simulink model "CementPlantVer1"  (R2019b)
settings: Solver=ode4  StartTime=0.0  StopTime=inf  FixedStep=0.01  RelTol=1e-3
(part 1 of 2)
settings Model: EnablePacing=on  Creator=huynh  LastModifiedBy=huynh

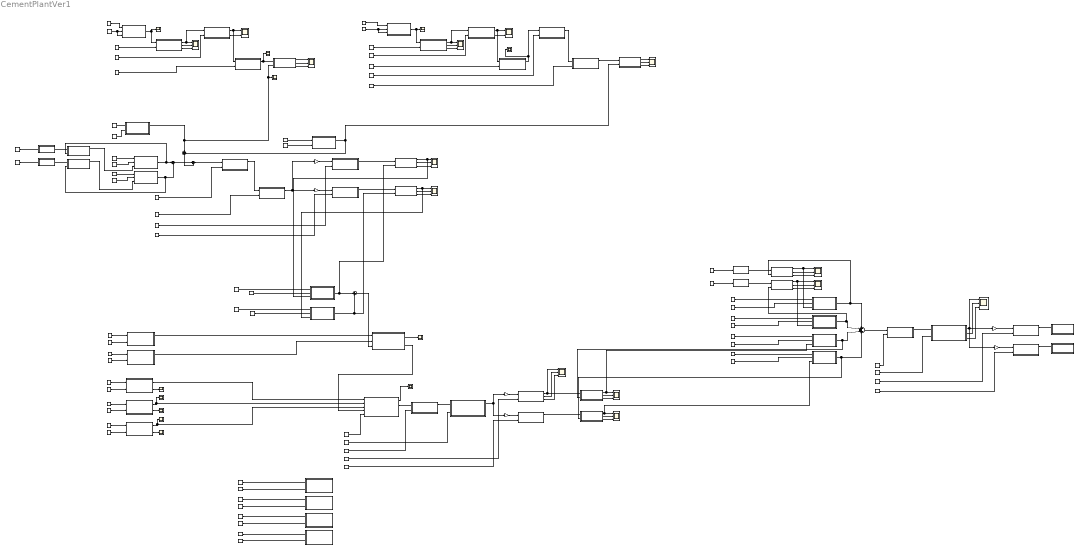
== system CementPlantVer1 ==
  note: CLAY AREA
  note: CementMill
  note: Fan System
  note: Clinker Area
  note: CoalMill
  note: RawMill
  note: Limestone Area
  note: Clay Area
  note: LIMESTONE AREA
  note: RAW MILL
  note: COAL MILL
  note: CLINKER AREA
  note: CEMENT MILL
  Additives Silo : Subsystem  mask{DensityOfMaterial=2.74, HighLevelSet=18, LowLevelSet=5, OutputGain=2}
      mask prompts: DensityOfMaterial "Density of material"; HighLevelSet "High Level"; LowLevelSet "Low Level"; OutputGain "Output Gain"
  Cement Silo 1 : Subsystem  mask{DensityOfMaterial=2.74, HighLevelSet=18, LowLevelSet=5, OutputGain=2}
      mask prompts: DensityOfMaterial "Density of material"; HighLevelSet "High Level"; LowLevelSet "Low Level"; OutputGain "Output Gain"
  Cement Silo 2 : Subsystem  mask{DensityOfMaterial=2.74, HighLevelSet=18, LowLevelSet=5, OutputGain=2}
      mask prompts: DensityOfMaterial "Density of material"; HighLevelSet "High Level"; LowLevelSet "Low Level"; OutputGain "Output Gain"
  CementMill Additives Valve In : Subsystem  mask{FlowConstant=400}
      mask prompts: FlowConstant "Flow Value"
  CementMill Additives Valve In Control : Constant
  CementMill Additives Valve Out : Subsystem  mask{OutputGain=100}
      mask prompts: OutputGain "Output Gian"
  CementMill Clinker Valve Out 1 : Subsystem  mask{OutputGain=200}
      mask prompts: OutputGain "Output Gian"
  CementMill Clinker Valve Out 2 : Subsystem  mask{OutputGain=200}
      mask prompts: OutputGain "Output Gian"
  CementMill Conveyor 1 : Subsystem
  CementMill Conveyor 2 : Subsystem
  CementMill Conveyor 3 : Subsystem
  CementMill Gypsum Valve In : Subsystem  mask{FlowConstant=400}
      mask prompts: FlowConstant "Flow Value"
  CementMill Gypsum Valve In Control : Constant
  CementMill Gypsum Valve Out : Subsystem  mask{OutputGain=100}
      mask prompts: OutputGain "Output Gian"
  CementMill Mix and Crusher : Subsystem
  Clay Conveyor 1 : Subsystem
  Clay Conveyor 2 : Subsystem
  Clay Crusher 1 : Subsystem
  Clay Storage : Subsystem  mask{DensityOfMaterial=2.74, HighLevelSet=18, LowLevelSet=5, OutputGain=2}
      mask prompts: DensityOfMaterial "Density of material"; HighLevelSet "High Level"; LowLevelSet "Low Level"; OutputGain "Output Gain"
  Clay Valve 1 : Subsystem  mask{OutputGain=400}
      mask prompts: OutputGain "Output Gian"
  Clinker Conveyor 1 : Subsystem
  Clinker Conveyor 2 : Subsystem
  Clinker Conveyor 3 : Subsystem
  Clinker Cooling Crusher : Subsystem
  Clinker Fan 1 : Subsystem
  Clinker Fan 2 : Subsystem
  Clinker Fan 3 : Subsystem
  Clinker Fan 4 : Subsystem
  Clinker In Valve 1 : Subsystem  mask{OutputGain=100}
      mask prompts: OutputGain "Output Gian"
  Clinker In Valve 2 : Subsystem  mask{OutputGain=100}
      mask prompts: OutputGain "Output Gian"
  Clinker PreHeater System : Subsystem
  Clinker PreHeater Temperature : Scope
  Clinker Rotary Kiln : Subsystem
  Clinker Rotary Kiln Temperature : Scope
  Clinker Silo 1 : Subsystem  mask{DensityOfMaterial=2.74, HighLevelSet=18, LowLevelSet=5, OutputGain=2}
      mask prompts: DensityOfMaterial "Density of material"; HighLevelSet "High Level"; LowLevelSet "Low Level"; OutputGain "Output Gain"
  Clinker Silo 2 : Subsystem  mask{DensityOfMaterial=2.74, HighLevelSet=18, LowLevelSet=5, OutputGain=2}
      mask prompts: DensityOfMaterial "Density of material"; HighLevelSet "High Level"; LowLevelSet "Low Level"; OutputGain "Output Gain"
  Clinker Valve Enable 1 : Constant
  Clinker Valve Enable 2 : Constant
  CoalMill Fan 1 : Subsystem
  CoalMill Pump 1 : Subsystem
  CoalMill Pump 2 : Subsystem
  CoalMill Pump 3 : Subsystem
  CoalMill Pump 4 : Subsystem
  Enable {1,3,7,9} (4 alike) : Constant
  Enable 5 : Constant  Value=0
  Enable CementMill Additives Valve Out : Constant
  Enable CementMill Clinker Valve Out 1 : Constant
  Enable CementMill Clinker Valve Out 2 : Constant  Value=0
  Enable CementMill Gypsum Valve Out : Constant
  Enable Clay Valve 1 : Constant
  Enable Clinker Fan {1..4} (4 alike) : Constant
  Enable Iron Valve 1 : Constant
  Enable Limestone Valve 1 : Constant
  Enable RawMill Conveyor 1 : Constant
  Enable RawMill Conveyor 2 : Constant
  Enable Sand Valve 1 : Constant
  F Input {1..5} (5 alike) : Constant  Value=50
  Frequence FB 1 : Scope
  Frequence FB 2 : Scope
  Frequence FB 3 : Scope
  Frequence In Clay Conveyor 1 : Constant  Value=50
  Frequence In Clay Conveyor 2 : Constant  Value=50
  Frequence In Clay Crusher 1 : Constant  Value=50
  Frequence In Limestone Conveyor 1 : Constant  Value=50
  Frequence In Limestone Conveyor 2 : Constant  Value=50
  Frequence In Limestone Conveyor 3 : Constant  Value=50
  Frequence In Limestone Crusher 1 : Constant  Value=50
  Frequence In Limestone Crusher 2 : Constant  Value=50
  Frequency In CementMill Conveyor 1 : Constant  Value=50
  Frequency In CementMill Conveyor 2 : Constant  Value=50
  Frequency In CementMill Conveyor 3 : Constant  Value=50
  Frequency In CementMill Mix and Crusher : Constant  Value=50
  Frequency In Clinker Conveyor 1 : Constant  Value=50
  Frequency In Clinker Conveyor 2 : Constant  Value=50
  Frequency In Clinker Conveyor 3 : Constant  Value=50
  Frequency In Clinker Cooling Crusher : Constant  Value=50
  Frequency In Clinker Fan {1..4} (4 alike) : Constant  Value=50
  Frequency In Clinker Rotary Kiln Frequence : Constant  Value=50
  Frequency In RawMill Conveyor {1..4} (4 alike) : Constant  Value=50
  Frequency In Roller Mill 1 : Constant  Value=50
  Gain{,1..5} (6 alike) : Gain  Gain=0.5
  Gypsum Silo : Subsystem  mask{DensityOfMaterial=2.74, HighLevelSet=18, LowLevelSet=5, OutputGain=2}
      mask prompts: DensityOfMaterial "Density of material"; HighLevelSet "High Level"; LowLevelSet "Low Level"; OutputGain "Output Gain"
  Input Frequency RawMill Conveyor 2 : Constant  Value=50
  Iron Silo : Subsystem  mask{DensityOfMaterial=2.74, HighLevelSet=18, LowLevelSet=5, OutputGain=2}
      mask prompts: DensityOfMaterial "Density of material"; HighLevelSet "High Level"; LowLevelSet "Low Level"; OutputGain "Output Gain"
  Limestone Conveyor 1 : Subsystem
  Limestone Conveyor 2 : Subsystem
  Limestone Conveyor 3 : Subsystem
  Limestone Crusher 1 : Subsystem
  Limestone Crusher 2 : Subsystem
  Limestone Storage : Subsystem  mask{DensityOfMaterial=2.74, HighLevelSet=18, LowLevelSet=5, OutputGain=2}
      mask prompts: DensityOfMaterial "Density of material"; HighLevelSet "High Level"; LowLevelSet "Low Level"; OutputGain "Output Gain"
  Limestone Valve 1 : Subsystem  mask{OutputGain=400}
      mask prompts: OutputGain "Output Gian"
  Output Test 2 : Scope
  Output Test 3 : Scope
  Percent Open CementMill Additives Valve Out : Constant  Value=100
  Percent Open CementMill Clinker Valve Out 1 : Constant  Value=100
  Percent Open CementMill Clinker Valve Out 2 : Constant  Value=100
  Percent Open CementMill Gypsum Valve Out : Constant  Value=100
  Percent Open Clay Valve 1 : Constant  Value=100
  Percent Open Clinker Valve 1 : Constant  Value=100
  Percent Open Clinker Valve 2 : Constant  Value=100
  Percent Open Iron Valve 1 : Constant  Value=100
  Percent Open Limestone Valve 1 : Constant  Value=100
  Percent Open Sand Valve 1 : Constant  Value=100
  RawMill Conveyor 1 : Subsystem  mask{OutputGain=100}
      mask prompts: OutputGain "Output Gain"
  RawMill Conveyor 2 : Subsystem  mask{OutputGain=100}
      mask prompts: OutputGain "Output Gain"
  RawMill Conveyor 3 : Subsystem
  RawMill Conveyor 4 : Subsystem
  RawMill Conveyor 5 : Subsystem
  RawMill Iron Valve In : Subsystem  mask{FlowConstant=300}
      mask prompts: FlowConstant "Flow Value"
  RawMill Iron Valve In Control : Constant
  RawMill Iron Valve Out : Subsystem  mask{OutputGain=100}
      mask prompts: OutputGain "Output Gian"
  RawMill Sand Valve In : Subsystem  mask{FlowConstant=300}
      mask prompts: FlowConstant "Flow Value"
  RawMill Sand Valve In Control : Constant
  RawMill Sand Valve Out : Subsystem  mask{OutputGain=100}
      mask prompts: OutputGain "Output Gian"
  RawMill Silo 1 : Subsystem  mask{DensityOfMaterial=2.74, HighLevelSet=18, LowLevelSet=5, OutputGain=2}
      mask prompts: DensityOfMaterial "Density of material"; HighLevelSet "High Level"; LowLevelSet "Low Level"; OutputGain "Output Gain"
  RawMill Silo 2 : Subsystem  mask{DensityOfMaterial=2.74, HighLevelSet=18, LowLevelSet=5, OutputGain=2}
      mask prompts: DensityOfMaterial "Density of material"; HighLevelSet "High Level"; LowLevelSet "Low Level"; OutputGain "Output Gain"
  Roller Mill 1 : Subsystem
  Sand Silo : Subsystem  mask{DensityOfMaterial=2.74, HighLevelSet=18, LowLevelSet=5, OutputGain=2}
      mask prompts: DensityOfMaterial "Density of material"; HighLevelSet "High Level"; LowLevelSet "Low Level"; OutputGain "Output Gain"
  Scope{1,3..4,6,9,11,13..18} (12 alike) : Scope  NumInputPorts=3
  Scope10 : Scope  NumInputPorts=2
  Scope12 : Scope
  Scope5 : Scope  NumInputPorts=2
  Scope7 : Scope
  Scope8 : Scope
  Sum{,1..3} (4 alike) : Sum  Inputs=|++
  Sum4 : Sum  Inputs=4
  Tốc độ đầu ra1 : Scope
  Tốc độ đầu ra2 : Scope
  wires:
  F Input 1/1 -> CoalMill Pump 1/1(Input Frequence)
  CoalMill Pump 1/2(Output Frequence) -> Frequence FB 1/1
  Enable 1/1 -> CoalMill Pump 1/2(Motor Enable)
  Enable RawMill Conveyor 1/1 -> RawMill Conveyor 1/2(Enable)
  Frequency In RawMill Conveyor 1/1 -> RawMill Conveyor 1/1(Input Frequence)
  RawMill Conveyor 1/1(Flow) -> Sum2/1, Clay Storage/2(Qout), Scope8/1
  F Input 2/1 -> CoalMill Pump 2/1(Input Frequence)
  CoalMill Pump 2/2(Output Frequence) -> Frequence FB 2/1
  CoalMill Pump 2/1(Output RPM) -> Tốc độ đầu ra1/1, Clinker Rotary Kiln/2(RPM In 2)
  Enable 3/1 -> CoalMill Pump 2/2(Motor Enable)
  Enable 5/1 -> CoalMill Pump 3/2(Motor Enable)
  CoalMill Pump 3/2(Output Frequence) -> Frequence FB 3/1
  CoalMill Pump 3/1(Output RPM) -> Clinker Rotary Kiln/3(RPM In 3), Tốc độ đầu ra2/1
  F Input 3/1 -> CoalMill Pump 3/1(Input Frequence)
  Percent Open Clay Valve 1/1 -> Clay Valve 1/1(Opening Percent)
  Enable Clay Valve 1/1 -> Clay Valve 1/3(Level of Silo), Clay Valve 1/2(Enable)
  Clay Valve 1/1(Flow) -> Clay Conveyor 1/1(Flow In), Output Test 2/1
  Frequence In Clay Conveyor 1/1 -> Clay Conveyor 1/2(Frequence In)
  Clay Conveyor 1/2(RPM out) -> Scope4/2
  Clay Conveyor 1/3(Frequence FB) -> Scope4/3
  Frequence In Clay Crusher 1/1 -> Clay Crusher 1/2(Frequence In)
  Clay Conveyor 1/1(Flow out) -> Clay Crusher 1/1(Flow In), Scope4/1
  Clay Crusher 1/1(Flow out) -> Clay Conveyor 2/1(Flow In), Scope5/1
  Clay Crusher 1/2(Frequence FB) -> Scope5/2
  Frequence In Clay Conveyor 2/1 -> Clay Conveyor 2/2(Frequence In)
  Clay Conveyor 2/1(Flow out) -> Scope7/1, Clay Storage/1(Qin)
  Clay Storage/3(Low) -> Scope6/3
  Clay Storage/2(High) -> Scope6/2
  Clay Storage/1(Level) -> Scope6/1
  Enable Limestone Valve 1/1 -> Limestone Valve 1/3(Level of Silo), Limestone Valve 1/2(Enable)
  Limestone Conveyor 1/2(RPM out) -> Scope9/2
  Limestone Storage/3(Low) -> Scope11/3
  Limestone Storage/1(Level) -> Scope11/1
  Frequence In Limestone Crusher 1/1 -> Limestone Crusher 1/2(Frequence In)
  Limestone Crusher 1/1(Flow out) -> Limestone Conveyor 2/1(Flow In), Scope10/1
  Limestone Crusher 1/2(Frequence FB) -> Scope10/2
  Limestone Storage/2(High) -> Scope11/2
  Limestone Valve 1/1(Flow) -> Limestone Conveyor 1/1(Flow In), Output Test 3/1
  Frequence In Limestone Conveyor 1/1 -> Limestone Conveyor 1/2(Frequence In)
  Limestone Conveyor 2/1(Flow out) -> Limestone Crusher 2/1(Flow In), Scope12/1
  Limestone Conveyor 1/3(Frequence FB) -> Scope9/3
  Limestone Conveyor 1/1(Flow out) -> Limestone Crusher 1/1(Flow In), Scope9/1
  Percent Open Limestone Valve 1/1 -> Limestone Valve 1/1(Opening Percent)
  Frequence In Limestone Conveyor 2/1 -> Limestone Conveyor 2/2(Frequence In)
  Frequence In Limestone Crusher 2/1 -> Limestone Crusher 2/2(Frequence In)
  Limestone Crusher 2/1(Flow out) -> Limestone Conveyor 3/1(Flow In)
  Frequence In Limestone Conveyor 3/1 -> Limestone Conveyor 3/2(Frequence In)
  Limestone Conveyor 3/1(Flow out) -> Limestone Storage/1(Qin)
  Input Frequency RawMill Conveyor 2/1 -> RawMill Conveyor 2/1(Input Frequence)
  Enable RawMill Conveyor 2/1 -> RawMill Conveyor 2/2(Enable)
  RawMill Conveyor 2/1(Flow) -> Sum2/2, Limestone Storage/2(Qout)
  Percent Open Sand Valve 1/1 -> RawMill Sand Valve Out/1(Opening Percent)
  Sum2/1 -> Sum3/2
  Sum1/1 -> Sum3/1
  Sum3/1 -> RawMill Conveyor 3/1(Flow In)
  Frequency In RawMill Conveyor 3/1 -> RawMill Conveyor 3/2(Frequence In)
  RawMill Conveyor 3/1(Flow out) -> Roller Mill 1/1(Flow In)
  Frequency In Roller Mill 1/1 -> Roller Mill 1/2(Frequence In)
  Roller Mill 1/1(Flow out) -> Gain1/1, Gain/1
  Frequency In RawMill Conveyor 4/1 -> RawMill Conveyor 4/2(Frequence In)
  RawMill Conveyor 4/1(Flow out) -> RawMill Silo 1/1(Qin)
  Gain/1 -> RawMill Conveyor 4/1(Flow In)
  Gain1/1 -> RawMill Conveyor 5/1(Flow In)
  RawMill Conveyor 5/1(Flow out) -> RawMill Silo 2/1(Qin)
  Frequency In RawMill Conveyor 2/1 -> RawMill Conveyor 5/2(Frequence In)
  Enable 7/1 -> CoalMill Pump 4/2(Motor Enable)
  F Input 4/1 -> CoalMill Pump 4/1(Input Frequence)
  F Input 5/1 -> CoalMill Fan 1/1(Input Frequence)
  Enable 9/1 -> CoalMill Fan 1/2(Motor Enable)
  CoalMill Pump 4/1(Output RPM) -> Clinker PreHeater System/1(RPM In 1)
  CoalMill Fan 1/1(Output RPM) -> Clinker PreHeater System/2(RPM In 2)
  CoalMill Pump 1/1(Output RPM) -> Clinker Rotary Kiln/1(RPM In 1)
  Gain2/1 -> Clinker Conveyor 2/1(Flow In)
  Clinker Cooling Crusher/1(Flow out) -> Gain3/1, Gain2/1
  Gain3/1 -> Clinker Conveyor 3/1(Flow In)
  Clinker PreHeater System/2(Flow out) -> Clinker Rotary Kiln/4(Flow In)
  Frequency In Clinker Rotary Kiln Frequence/1 -> Clinker Rotary Kiln/5(Rotary Kiln Frequence)
  Frequency In Clinker Cooling Crusher/1 -> Clinker Cooling Crusher/2(Frequence In)
  Clinker Rotary Kiln/1(Temperature) -> Clinker Rotary Kiln Temperature/1
  Clinker PreHeater System/1(Temperature) -> Clinker PreHeater Temperature/1
  Clinker Conveyor 2/1(Flow out) -> Clinker Silo 1/1(Qin), Scope1/1
  Clinker Conveyor 2/2(RPM out) -> Scope1/2
  Clinker Conveyor 2/3(Frequence FB) -> Scope1/3
  Sum/1 -> Clinker PreHeater System/3(Flow In)
  Clinker Conveyor 3/1(Flow out) -> Clinker Silo 2/1(Qin)
  Clinker In Valve 2/1(Flow) -> RawMill Silo 2/2(Qout), Sum/2
  Clinker In Valve 1/1(Flow) -> RawMill Silo 1/2(Qout), Sum/1
  Percent Open Clinker Valve 1/1 -> Clinker In Valve 1/1(Opening Percent)
  Percent Open Clinker Valve 2/1 -> Clinker In Valve 2/1(Opening Percent)
  Clinker Valve Enable 1/1 -> Clinker In Valve 1/2(Enable)
  Clinker Valve Enable 2/1 -> Clinker In Valve 2/2(Enable)
  RawMill Silo 1/1(Level) -> Clinker In Valve 1/3(Level of Silo), Scope3/1
  RawMill Silo 2/1(Level) -> Scope13/1, Clinker In Valve 2/3(Level of Silo)
  RawMill Silo 1/3(Low) -> Scope3/3
  RawMill Silo 1/2(High) -> Scope3/2
  RawMill Silo 2/2(High) -> Scope13/2
  RawMill Silo 2/3(Low) -> Scope13/3
  Clinker Silo 1/1(Level) -> CementMill Clinker Valve Out 1/3(Level of Silo), Scope14/1
  Clinker Silo 1/2(High) -> Scope14/2
  Clinker Silo 1/3(Low) -> Scope14/3
  Clinker Silo 2/1(Level) -> CementMill Clinker Valve Out 2/3(Level of Silo), Scope15/1
  Clinker Silo 2/2(High) -> Scope15/2
  Clinker Silo 2/3(Low) -> Scope15/3
  Clinker Rotary Kiln/2(Flow Out) -> Clinker Conveyor 1/1(Flow In)
  Clinker Conveyor 1/1(Flow out) -> Clinker Cooling Crusher/1(Flow In)
  Frequency In Clinker Conveyor 1/1 -> Clinker Conveyor 1/2(Frequence In)
  Frequency In Clinker Conveyor 2/1 -> Clinker Conveyor 2/2(Frequence In)
  Frequency In Clinker Conveyor 3/1 -> Clinker Conveyor 3/2(Frequence In)
  Frequency In Clinker Fan 1/1 -> Clinker Fan 1/1(Input Frequence)
  Frequency In Clinker Fan 2/1 -> Clinker Fan 2/1(Input Frequence)
  Frequency In Clinker Fan 3/1 -> Clinker Fan 3/1(Input Frequence)
  Frequency In Clinker Fan 4/1 -> Clinker Fan 4/1(Input Frequence)
  Enable Clinker Fan 1/1 -> Clinker Fan 1/2(Motor Enable)
  Enable Clinker Fan 2/1 -> Clinker Fan 2/2(Motor Enable)
  Enable Clinker Fan 3/1 -> Clinker Fan 3/2(Motor Enable)
  Enable Clinker Fan 4/1 -> Clinker Fan 4/2(Motor Enable)
  CementMill Gypsum Valve Out/1(Flow) -> Gypsum Silo/2(Qout), Sum4/1
  CementMill Additives Valve Out/1(Flow) -> Additives Silo/2(Qout), Sum4/2
  CementMill Clinker Valve Out 1/1(Flow) -> Clinker Silo 1/2(Qout), Sum4/3
  CementMill Clinker Valve Out 2/1(Flow) -> Clinker Silo 2/2(Qout), Sum4/4
  Sum4/1 -> CementMill Conveyor 1/1(Flow In)
  Percent Open CementMill Clinker Valve Out 1/1 -> CementMill Clinker Valve Out 1/1(Opening Percent)
  Percent Open CementMill Clinker Valve Out 2/1 -> CementMill Clinker Valve Out 2/1(Opening Percent)
  Enable CementMill Clinker Valve Out 1/1 -> CementMill Clinker Valve Out 1/2(Enable)
  Enable CementMill Clinker Valve Out 2/1 -> CementMill Clinker Valve Out 2/2(Enable)
  Frequency In CementMill Conveyor 1/1 -> CementMill Conveyor 1/2(Frequence In)
  CementMill Conveyor 1/1(Flow out) -> CementMill Mix and Crusher/1(Flow In)
  Frequency In CementMill Mix and Crusher/1 -> CementMill Mix and Crusher/2(Frequence In)
  CementMill Gypsum Valve In/1(Flow Out) -> Gypsum Silo/1(Qin)
  CementMill Gypsum Valve In Control/1 -> CementMill Gypsum Valve In/1(Open/Close)
  Gypsum Silo/1(Level) -> Scope16/1, CementMill Gypsum Valve Out/3(Level of Silo)
  Percent Open CementMill Gypsum Valve Out/1 -> CementMill Gypsum Valve Out/1(Opening Percent)
  Percent Open CementMill Additives Valve Out/1 -> CementMill Additives Valve Out/1(Opening Percent)
  Enable CementMill Gypsum Valve Out/1 -> CementMill Gypsum Valve Out/2(Enable)
  Enable CementMill Additives Valve Out/1 -> CementMill Additives Valve Out/2(Enable)
  Additives Silo/1(Level) -> Scope17/1, CementMill Additives Valve Out/3(Level of Silo)
  CementMill Additives Valve In Control/1 -> CementMill Additives Valve In/1(Open/Close)
  CementMill Additives Valve In/1(Flow Out) -> Additives Silo/1(Qin)
  Gypsum Silo/2(High) -> Scope16/2
  Gypsum Silo/3(Low) -> Scope16/3
  Additives Silo/3(Low) -> Scope17/3
  Additives Silo/2(High) -> Scope17/2
  CementMill Mix and Crusher/2(RPM out) -> Scope18/2
  CementMill Mix and Crusher/1(Flow out) -> Scope18/1, Gain5/1, Gain4/1
  CementMill Mix and Crusher/3(Frequence FB) -> Scope18/3
  Gain4/1 -> CementMill Conveyor 2/1(Flow In)
  Gain5/1 -> CementMill Conveyor 3/1(Flow In)
  CementMill Conveyor 2/1(Flow out) -> Cement Silo 1/1(Qin)
  Frequency In CementMill Conveyor 2/1 -> CementMill Conveyor 2/2(Frequence In)
  Frequency In CementMill Conveyor 3/1 -> CementMill Conveyor 3/2(Frequence In)
  CementMill Conveyor 3/1(Flow out) -> Cement Silo 2/1(Qin)
  RawMill Iron Valve In Control/1 -> RawMill Iron Valve In/1(Open/Close)
  RawMill Sand Valve In Control/1 -> RawMill Sand Valve In/1(Open/Close)
  RawMill Iron Valve In/1(Flow Out) -> Iron Silo/1(Qin)
  RawMill Sand Valve In/1(Flow Out) -> Sand Silo/1(Qin)
  RawMill Sand Valve Out/1(Flow) -> Sand Silo/2(Qout), Sum1/1
  Enable Sand Valve 1/1 -> RawMill Sand Valve Out/2(Enable)
  Sand Silo/1(Level) -> RawMill Sand Valve Out/3(Level of Silo)
  RawMill Iron Valve Out/1(Flow) -> Iron Silo/2(Qout), Sum1/2
  Percent Open Iron Valve 1/1 -> RawMill Iron Valve Out/1(Opening Percent)
  Enable Iron Valve 1/1 -> RawMill Iron Valve Out/2(Enable)
  Iron Silo/1(Level) -> RawMill Iron Valve Out/3(Level of Silo)

== system CementPlantVer1/Additives Silo ==
  Qin : Inport
  Qout : Inport  Port=2
  A : Gain  Gain=1/(3.14*3*3)
  Convert h to s : Constant  Value=3600
  Density of Clay : Constant  Value=DensityOfMaterial
  Divide : Product  Inputs=*/
  Divide1 : Product  Inputs=*/
  High Operator : RelationalOperator  OutDataTypeStr=boolean  RndMeth=Simplest
  High Level Set (m) : Constant  Value=HighLevelSet
  Low Operator : RelationalOperator  Operator=<=  OutDataTypeStr=boolean  RndMeth=Simplest
  Low Level Set (m) : Constant  Value=LowLevelSet
  Output Coefficient : Gain  Gain=OutputGain
  Saturation Limit : Saturate  UpperLimit=20  LowerLimit=0
  Sum1 : Sum  Inputs=|+-
  Transfer Fnc of Silo : TransferFcn  Denominator=[1 0]
  Level : Outport
  High : Outport  Port=2
  Low : Outport  Port=3
  wires:
  A/1 -> Output Coefficient/1
  Low Operator/1 -> Low/1
  High Level Set (m)/1 -> High Operator/2
  Low Level Set (m)/1 -> Low Operator/2
  Density of Clay/1 -> Divide/2
  Output Coefficient/1 -> Saturation Limit/1
  Convert h to s/1 -> Divide1/2
  Transfer Fnc of Silo/1 -> A/1
  Divide1/1 -> Transfer Fnc of Silo/1
  High Operator/1 -> High/1
  Saturation Limit/1 -> Level/1, Low Operator/1, High Operator/1
  Divide/1 -> Divide1/1
  Sum1/1 -> Divide/1
  Qin/1 -> Sum1/1
  Qout/1 -> Sum1/2

== system CementPlantVer1/Cement Silo 1 ==
  Qin : Inport
  Qout : Inport  Port=2
  A : Gain  Gain=1/(3.14*3*3)
  Convert h to s : Constant  Value=3600
  Density of Clay : Constant  Value=DensityOfMaterial
  Divide : Product  Inputs=*/
  Divide1 : Product  Inputs=*/
  High Operator : RelationalOperator  OutDataTypeStr=boolean  RndMeth=Simplest
  High Level Set (m) : Constant  Value=HighLevelSet
  Low Operator : RelationalOperator  Operator=<=  OutDataTypeStr=boolean  RndMeth=Simplest
  Low Level Set (m) : Constant  Value=LowLevelSet
  Output Coefficient : Gain  Gain=OutputGain
  Saturation Limit : Saturate  UpperLimit=20  LowerLimit=0
  Sum1 : Sum  Inputs=|+-
  Transfer Fnc of Silo : TransferFcn  Denominator=[1 0]
  Level : Outport
  High : Outport  Port=2
  Low : Outport  Port=3
  wires:
  A/1 -> Output Coefficient/1
  Low Operator/1 -> Low/1
  High Level Set (m)/1 -> High Operator/2
  Low Level Set (m)/1 -> Low Operator/2
  Density of Clay/1 -> Divide/2
  Output Coefficient/1 -> Saturation Limit/1
  Convert h to s/1 -> Divide1/2
  Transfer Fnc of Silo/1 -> A/1
  Divide1/1 -> Transfer Fnc of Silo/1
  High Operator/1 -> High/1
  Saturation Limit/1 -> Level/1, Low Operator/1, High Operator/1
  Divide/1 -> Divide1/1
  Sum1/1 -> Divide/1
  Qin/1 -> Sum1/1
  Qout/1 -> Sum1/2

== system CementPlantVer1/Cement Silo 2 ==
  Qin : Inport
  Qout : Inport  Port=2
  A : Gain  Gain=1/(3.14*3*3)
  Convert h to s : Constant  Value=3600
  Density of Clay : Constant  Value=DensityOfMaterial
  Divide : Product  Inputs=*/
  Divide1 : Product  Inputs=*/
  High Operator : RelationalOperator  OutDataTypeStr=boolean  RndMeth=Simplest
  High Level Set (m) : Constant  Value=HighLevelSet
  Low Operator : RelationalOperator  Operator=<=  OutDataTypeStr=boolean  RndMeth=Simplest
  Low Level Set (m) : Constant  Value=LowLevelSet
  Output Coefficient : Gain  Gain=OutputGain
  Saturation Limit : Saturate  UpperLimit=20  LowerLimit=0
  Sum1 : Sum  Inputs=|+-
  Transfer Fnc of Silo : TransferFcn  Denominator=[1 0]
  Level : Outport
  High : Outport  Port=2
  Low : Outport  Port=3
  wires:
  A/1 -> Output Coefficient/1
  Low Operator/1 -> Low/1
  High Level Set (m)/1 -> High Operator/2
  Low Level Set (m)/1 -> Low Operator/2
  Density of Clay/1 -> Divide/2
  Output Coefficient/1 -> Saturation Limit/1
  Convert h to s/1 -> Divide1/2
  Transfer Fnc of Silo/1 -> A/1
  Divide1/1 -> Transfer Fnc of Silo/1
  High Operator/1 -> High/1
  Saturation Limit/1 -> Level/1, Low Operator/1, High Operator/1
  Divide/1 -> Divide1/1
  Sum1/1 -> Divide/1
  Qin/1 -> Sum1/1
  Qout/1 -> Sum1/2

== system CementPlantVer1/CementMill Additives Valve In ==
  Open/Close : Inport
  Constant : Constant  Value=0
  Constant1 : Constant  Value=FlowConstant
  Switch : Switch  Threshold=1
  Transfer Fcn : TransferFcn  Denominator=[0.5 1]
  Flow Out : Outport
  wires:
  Open/Close/1 -> Switch/2
  Constant/1 -> Switch/3
  Constant1/1 -> Switch/1
  Switch/1 -> Transfer Fcn/1
  Transfer Fcn/1 -> Flow Out/1

== system CementPlantVer1/CementMill Additives Valve Out ==
  Opening Percent : Inport
  Enable : Inport  Port=2
  Level of Silo : Inport  Port=3
  Constant : Constant  Value=0
  Delay 1s : TransportDelay
  Divide : Product  Inputs=*/
  Maxium Value : Constant  Value=100
  Output Coefficient : Gain  Gain=OutputGain
  Switch : Switch  Threshold=1
  Switch1 : Switch  Criteria=u2 > Threshold
  Transfer Fnc : TransferFcn  Denominator=[20 1]
  Flow : Outport
  wires:
  Transfer Fnc/1 -> Delay 1s/1
  Enable/1 -> Switch/2
  Constant/1 -> Switch/3, Switch1/3
  Opening Percent/1 -> Divide/1
  Divide/1 -> Switch/1
  Maxium Value/1 -> Divide/2
  Output Coefficient/1 -> Flow/1
  Delay 1s/1 -> Output Coefficient/1
  Switch1/1 -> Transfer Fnc/1
  Switch/1 -> Switch1/1
  Level of Silo/1 -> Switch1/2

== system CementPlantVer1/CementMill Clinker Valve Out 1 ==
  Opening Percent : Inport
  Enable : Inport  Port=2
  Level of Silo : Inport  Port=3
  Constant : Constant  Value=0
  Delay 1s : TransportDelay
  Divide : Product  Inputs=*/
  Maxium Value : Constant  Value=100
  Output Coefficient : Gain  Gain=OutputGain
  Switch : Switch  Threshold=1
  Switch1 : Switch  Criteria=u2 > Threshold
  Transfer Fnc : TransferFcn  Denominator=[20 1]
  Flow : Outport
  wires:
  Transfer Fnc/1 -> Delay 1s/1
  Enable/1 -> Switch/2
  Constant/1 -> Switch/3, Switch1/3
  Opening Percent/1 -> Divide/1
  Divide/1 -> Switch/1
  Maxium Value/1 -> Divide/2
  Output Coefficient/1 -> Flow/1
  Delay 1s/1 -> Output Coefficient/1
  Switch1/1 -> Transfer Fnc/1
  Switch/1 -> Switch1/1
  Level of Silo/1 -> Switch1/2

== system CementPlantVer1/CementMill Clinker Valve Out 2 ==
  Opening Percent : Inport
  Enable : Inport  Port=2
  Level of Silo : Inport  Port=3
  Constant : Constant  Value=0
  Delay 1s : TransportDelay
  Divide : Product  Inputs=*/
  Maxium Value : Constant  Value=100
  Output Coefficient : Gain  Gain=OutputGain
  Switch : Switch  Threshold=1
  Switch1 : Switch  Criteria=u2 > Threshold
  Transfer Fnc : TransferFcn  Denominator=[20 1]
  Flow : Outport
  wires:
  Transfer Fnc/1 -> Delay 1s/1
  Enable/1 -> Switch/2
  Constant/1 -> Switch/3, Switch1/3
  Opening Percent/1 -> Divide/1
  Divide/1 -> Switch/1
  Maxium Value/1 -> Divide/2
  Output Coefficient/1 -> Flow/1
  Delay 1s/1 -> Output Coefficient/1
  Switch1/1 -> Transfer Fnc/1
  Switch/1 -> Switch1/1
  Level of Silo/1 -> Switch1/2

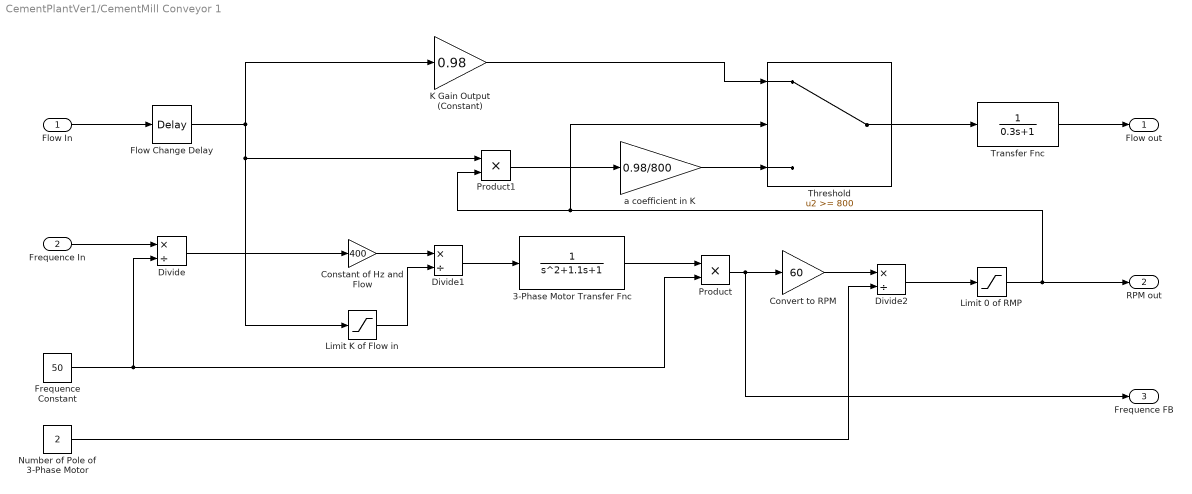
== system CementPlantVer1/CementMill Conveyor 1 ==
  Flow In : Inport
  Frequence In : Inport  Port=2
  3-Phase Motor Transfer Fnc : TransferFcn  Denominator=[1 1.1 1]
  Constant of Hz and Flow : Gain  Gain=400
  Convert to RPM : Gain  Gain=60
  Divide : Product  Inputs=*/
  Divide1 : Product  Inputs=*/
  Divide2 : Product  Inputs=*/
  Flow Change Delay : TransportDelay  DelayTime=0.5
  Frequence Constant : Constant  Value=50
  K Gain Output (Constant) : Gain  Gain=0.98
  Limit 0 of RMP : Saturate  UpperLimit=inf  LowerLimit=0
  Limit K of Flow in : Saturate  UpperLimit=inf  LowerLimit=400
  Number of Pole of 3-Phase Motor : Constant  Value=2
  Product : Product
  Product1 : Product
  Threshold : Switch  Threshold=800
  Transfer Fnc : TransferFcn  Denominator=[0.3 1]
  a coefficient in K : Gain  Gain=0.98/800
  Flow out : Outport
  RPM out : Outport  Port=2
  Frequence FB : Outport  Port=3
  wires:
  Constant of Hz and Flow/1 -> Divide1/1
  Limit K of Flow in/1 -> Divide1/2
  Divide1/1 -> 3-Phase Motor Transfer Fnc/1
  Limit 0 of RMP/1 -> RPM out/1, Threshold/2, Product1/2
  Flow In/1 -> Flow Change Delay/1
  Flow Change Delay/1 -> Product1/1, Limit K of Flow in/1, K Gain Output (Constant)/1
  K Gain Output (Constant)/1 -> Threshold/1
  Frequence In/1 -> Divide/1
  Divide/1 -> Constant of Hz and Flow/1
  Frequence Constant/1 -> Product/2, Divide/2
  3-Phase Motor Transfer Fnc/1 -> Product/1
  Product/1 -> Frequence FB/1, Convert to RPM/1
  Convert to RPM/1 -> Divide2/1
  Divide2/1 -> Limit 0 of RMP/1
  Number of Pole of 3-Phase Motor/1 -> Divide2/2
  Threshold/1 -> Transfer Fnc/1
  Transfer Fnc/1 -> Flow out/1
  Product1/1 -> a coefficient in K/1
  a coefficient in K/1 -> Threshold/3

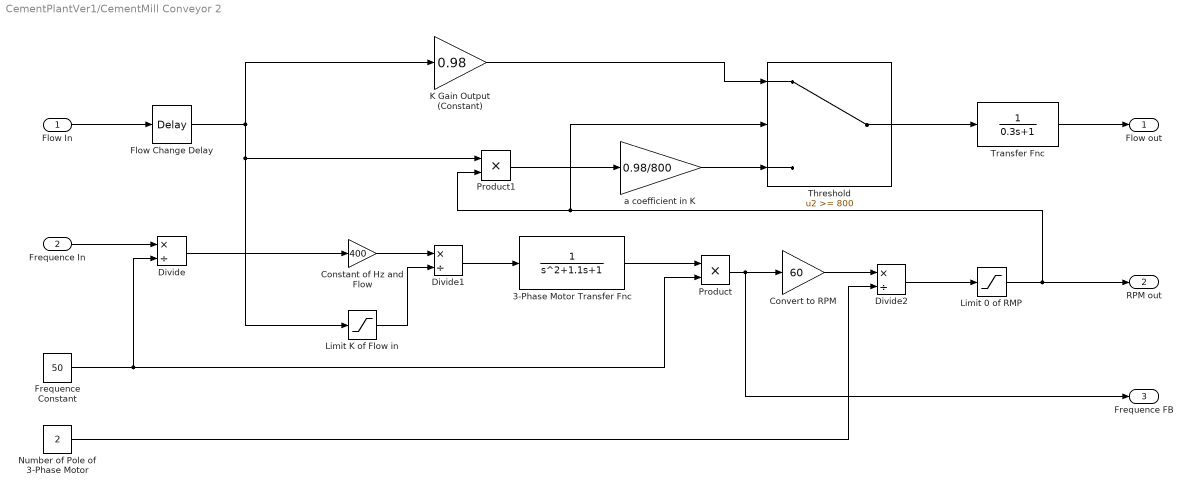
== system CementPlantVer1/CementMill Conveyor 2 ==
  Flow In : Inport
  Frequence In : Inport  Port=2
  3-Phase Motor Transfer Fnc : TransferFcn  Denominator=[1 1.1 1]
  Constant of Hz and Flow : Gain  Gain=400
  Convert to RPM : Gain  Gain=60
  Divide : Product  Inputs=*/
  Divide1 : Product  Inputs=*/
  Divide2 : Product  Inputs=*/
  Flow Change Delay : TransportDelay  DelayTime=0.5
  Frequence Constant : Constant  Value=50
  K Gain Output (Constant) : Gain  Gain=0.98
  Limit 0 of RMP : Saturate  UpperLimit=inf  LowerLimit=0
  Limit K of Flow in : Saturate  UpperLimit=inf  LowerLimit=400
  Number of Pole of 3-Phase Motor : Constant  Value=2
  Product : Product
  Product1 : Product
  Threshold : Switch  Threshold=800
  Transfer Fnc : TransferFcn  Denominator=[0.3 1]
  a coefficient in K : Gain  Gain=0.98/800
  Flow out : Outport
  RPM out : Outport  Port=2
  Frequence FB : Outport  Port=3
  wires:
  Constant of Hz and Flow/1 -> Divide1/1
  Limit K of Flow in/1 -> Divide1/2
  Divide1/1 -> 3-Phase Motor Transfer Fnc/1
  Limit 0 of RMP/1 -> RPM out/1, Threshold/2, Product1/2
  Flow In/1 -> Flow Change Delay/1
  Flow Change Delay/1 -> Product1/1, Limit K of Flow in/1, K Gain Output (Constant)/1
  K Gain Output (Constant)/1 -> Threshold/1
  Frequence In/1 -> Divide/1
  Divide/1 -> Constant of Hz and Flow/1
  Frequence Constant/1 -> Product/2, Divide/2
  3-Phase Motor Transfer Fnc/1 -> Product/1
  Product/1 -> Frequence FB/1, Convert to RPM/1
  Convert to RPM/1 -> Divide2/1
  Divide2/1 -> Limit 0 of RMP/1
  Number of Pole of 3-Phase Motor/1 -> Divide2/2
  Threshold/1 -> Transfer Fnc/1
  Transfer Fnc/1 -> Flow out/1
  Product1/1 -> a coefficient in K/1
  a coefficient in K/1 -> Threshold/3

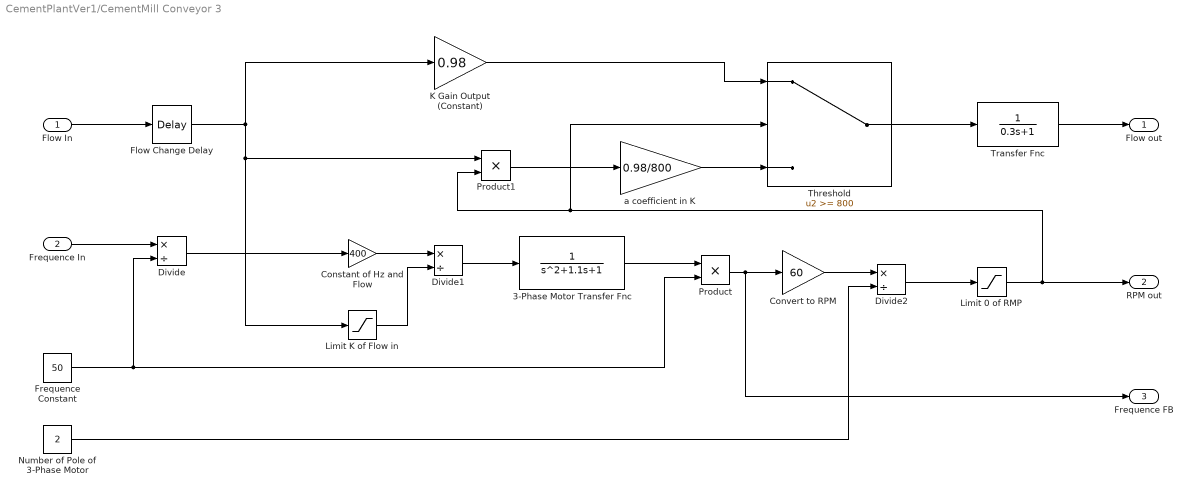
== system CementPlantVer1/CementMill Conveyor 3 ==
  Flow In : Inport
  Frequence In : Inport  Port=2
  3-Phase Motor Transfer Fnc : TransferFcn  Denominator=[1 1.1 1]
  Constant of Hz and Flow : Gain  Gain=400
  Convert to RPM : Gain  Gain=60
  Divide : Product  Inputs=*/
  Divide1 : Product  Inputs=*/
  Divide2 : Product  Inputs=*/
  Flow Change Delay : TransportDelay  DelayTime=0.5
  Frequence Constant : Constant  Value=50
  K Gain Output (Constant) : Gain  Gain=0.98
  Limit 0 of RMP : Saturate  UpperLimit=inf  LowerLimit=0
  Limit K of Flow in : Saturate  UpperLimit=inf  LowerLimit=400
  Number of Pole of 3-Phase Motor : Constant  Value=2
  Product : Product
  Product1 : Product
  Threshold : Switch  Threshold=800
  Transfer Fnc : TransferFcn  Denominator=[0.3 1]
  a coefficient in K : Gain  Gain=0.98/800
  Flow out : Outport
  RPM out : Outport  Port=2
  Frequence FB : Outport  Port=3
  wires:
  Constant of Hz and Flow/1 -> Divide1/1
  Limit K of Flow in/1 -> Divide1/2
  Divide1/1 -> 3-Phase Motor Transfer Fnc/1
  Limit 0 of RMP/1 -> RPM out/1, Threshold/2, Product1/2
  Flow In/1 -> Flow Change Delay/1
  Flow Change Delay/1 -> Product1/1, Limit K of Flow in/1, K Gain Output (Constant)/1
  K Gain Output (Constant)/1 -> Threshold/1
  Frequence In/1 -> Divide/1
  Divide/1 -> Constant of Hz and Flow/1
  Frequence Constant/1 -> Product/2, Divide/2
  3-Phase Motor Transfer Fnc/1 -> Product/1
  Product/1 -> Frequence FB/1, Convert to RPM/1
  Convert to RPM/1 -> Divide2/1
  Divide2/1 -> Limit 0 of RMP/1
  Number of Pole of 3-Phase Motor/1 -> Divide2/2
  Threshold/1 -> Transfer Fnc/1
  Transfer Fnc/1 -> Flow out/1
  Product1/1 -> a coefficient in K/1
  a coefficient in K/1 -> Threshold/3

== system CementPlantVer1/CementMill Gypsum Valve In ==
  Open/Close : Inport
  Constant : Constant  Value=0
  Constant1 : Constant  Value=FlowConstant
  Switch : Switch  Threshold=1
  Transfer Fcn : TransferFcn  Denominator=[0.5 1]
  Flow Out : Outport
  wires:
  Open/Close/1 -> Switch/2
  Constant/1 -> Switch/3
  Constant1/1 -> Switch/1
  Switch/1 -> Transfer Fcn/1
  Transfer Fcn/1 -> Flow Out/1

== system CementPlantVer1/CementMill Gypsum Valve Out ==
  Opening Percent : Inport
  Enable : Inport  Port=2
  Level of Silo : Inport  Port=3
  Constant : Constant  Value=0
  Delay 1s : TransportDelay
  Divide : Product  Inputs=*/
  Maxium Value : Constant  Value=100
  Output Coefficient : Gain  Gain=OutputGain
  Switch : Switch  Threshold=1
  Switch1 : Switch  Criteria=u2 > Threshold
  Transfer Fnc : TransferFcn  Denominator=[20 1]
  Flow : Outport
  wires:
  Transfer Fnc/1 -> Delay 1s/1
  Enable/1 -> Switch/2
  Constant/1 -> Switch/3, Switch1/3
  Opening Percent/1 -> Divide/1
  Divide/1 -> Switch/1
  Maxium Value/1 -> Divide/2
  Output Coefficient/1 -> Flow/1
  Delay 1s/1 -> Output Coefficient/1
  Switch1/1 -> Transfer Fnc/1
  Switch/1 -> Switch1/1
  Level of Silo/1 -> Switch1/2

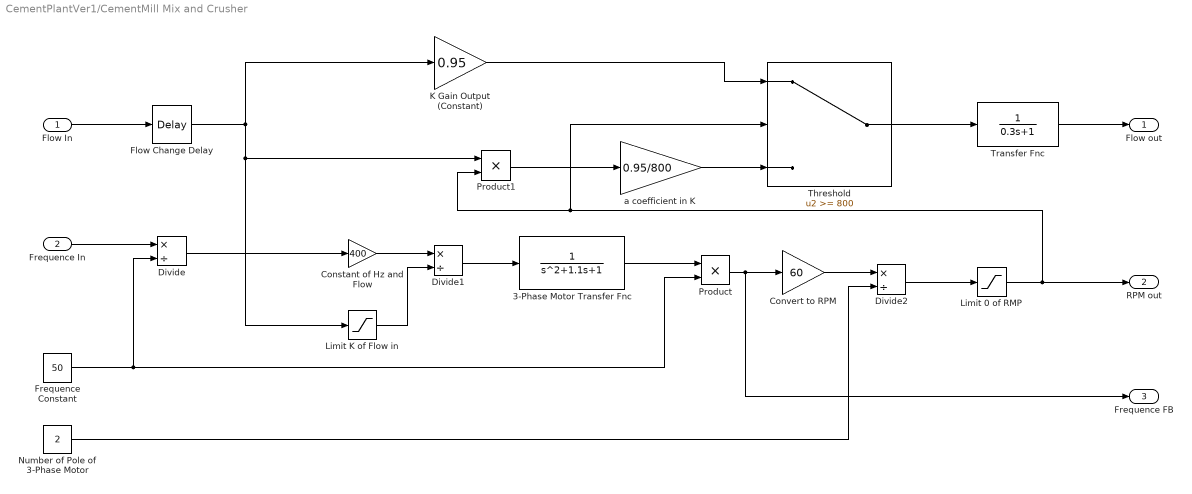
== system CementPlantVer1/CementMill Mix and Crusher ==
  Flow In : Inport
  Frequence In : Inport  Port=2
  3-Phase Motor Transfer Fnc : TransferFcn  Denominator=[1 1.1 1]
  Constant of Hz and Flow : Gain  Gain=400
  Convert to RPM : Gain  Gain=60
  Divide : Product  Inputs=*/
  Divide1 : Product  Inputs=*/
  Divide2 : Product  Inputs=*/
  Flow Change Delay : TransportDelay  DelayTime=0.5
  Frequence Constant : Constant  Value=50
  K Gain Output (Constant) : Gain  Gain=0.95
  Limit 0 of RMP : Saturate  UpperLimit=inf  LowerLimit=0
  Limit K of Flow in : Saturate  UpperLimit=inf  LowerLimit=400
  Number of Pole of 3-Phase Motor : Constant  Value=2
  Product : Product
  Product1 : Product
  Threshold : Switch  Threshold=800
  Transfer Fnc : TransferFcn  Denominator=[0.3 1]
  a coefficient in K : Gain  Gain=0.95/800
  Flow out : Outport
  RPM out : Outport  Port=2
  Frequence FB : Outport  Port=3
  wires:
  Constant of Hz and Flow/1 -> Divide1/1
  Limit K of Flow in/1 -> Divide1/2
  Divide1/1 -> 3-Phase Motor Transfer Fnc/1
  Limit 0 of RMP/1 -> RPM out/1, Threshold/2, Product1/2
  Flow In/1 -> Flow Change Delay/1
  Flow Change Delay/1 -> Product1/1, Limit K of Flow in/1, K Gain Output (Constant)/1
  K Gain Output (Constant)/1 -> Threshold/1
  Frequence In/1 -> Divide/1
  Divide/1 -> Constant of Hz and Flow/1
  Frequence Constant/1 -> Product/2, Divide/2
  3-Phase Motor Transfer Fnc/1 -> Product/1
  Product/1 -> Frequence FB/1, Convert to RPM/1
  Convert to RPM/1 -> Divide2/1
  Divide2/1 -> Limit 0 of RMP/1
  Number of Pole of 3-Phase Motor/1 -> Divide2/2
  Threshold/1 -> Transfer Fnc/1
  Transfer Fnc/1 -> Flow out/1
  Product1/1 -> a coefficient in K/1
  a coefficient in K/1 -> Threshold/3

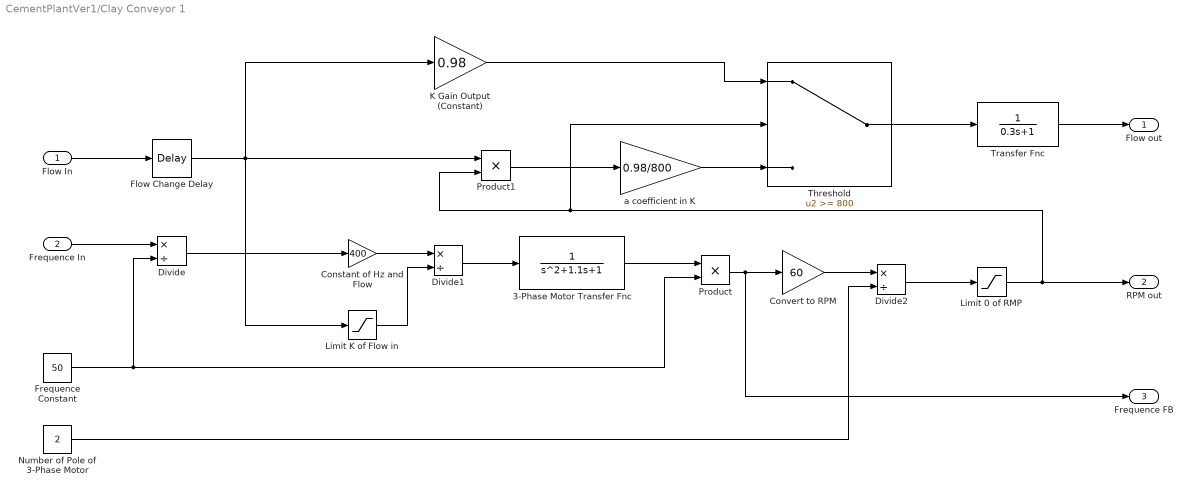
== system CementPlantVer1/Clay Conveyor 1 ==
  Flow In : Inport
  Frequence In : Inport  Port=2
  3-Phase Motor Transfer Fnc : TransferFcn  Denominator=[1 1.1 1]
  Constant of Hz and Flow : Gain  Gain=400
  Convert to RPM : Gain  Gain=60
  Divide : Product  Inputs=*/
  Divide1 : Product  Inputs=*/
  Divide2 : Product  Inputs=*/
  Flow Change Delay : TransportDelay  DelayTime=0.5
  Frequence Constant : Constant  Value=50
  K Gain Output (Constant) : Gain  Gain=0.98
  Limit 0 of RMP : Saturate  UpperLimit=inf  LowerLimit=0
  Limit K of Flow in : Saturate  UpperLimit=inf  LowerLimit=400
  Number of Pole of 3-Phase Motor : Constant  Value=2
  Product : Product
  Product1 : Product
  Threshold : Switch  Threshold=800
  Transfer Fnc : TransferFcn  Denominator=[0.3 1]
  a coefficient in K : Gain  Gain=0.98/800
  Flow out : Outport
  RPM out : Outport  Port=2
  Frequence FB : Outport  Port=3
  wires:
  Constant of Hz and Flow/1 -> Divide1/1
  Limit K of Flow in/1 -> Divide1/2
  Divide1/1 -> 3-Phase Motor Transfer Fnc/1
  Limit 0 of RMP/1 -> RPM out/1, Threshold/2, Product1/2
  Flow In/1 -> Flow Change Delay/1
  Flow Change Delay/1 -> K Gain Output (Constant)/1, Product1/1, Limit K of Flow in/1
  K Gain Output (Constant)/1 -> Threshold/1
  Frequence In/1 -> Divide/1
  Divide/1 -> Constant of Hz and Flow/1
  Frequence Constant/1 -> Product/2, Divide/2
  3-Phase Motor Transfer Fnc/1 -> Product/1
  Product/1 -> Frequence FB/1, Convert to RPM/1
  Convert to RPM/1 -> Divide2/1
  Divide2/1 -> Limit 0 of RMP/1
  Number of Pole of 3-Phase Motor/1 -> Divide2/2
  Threshold/1 -> Transfer Fnc/1
  Transfer Fnc/1 -> Flow out/1
  Product1/1 -> a coefficient in K/1
  a coefficient in K/1 -> Threshold/3

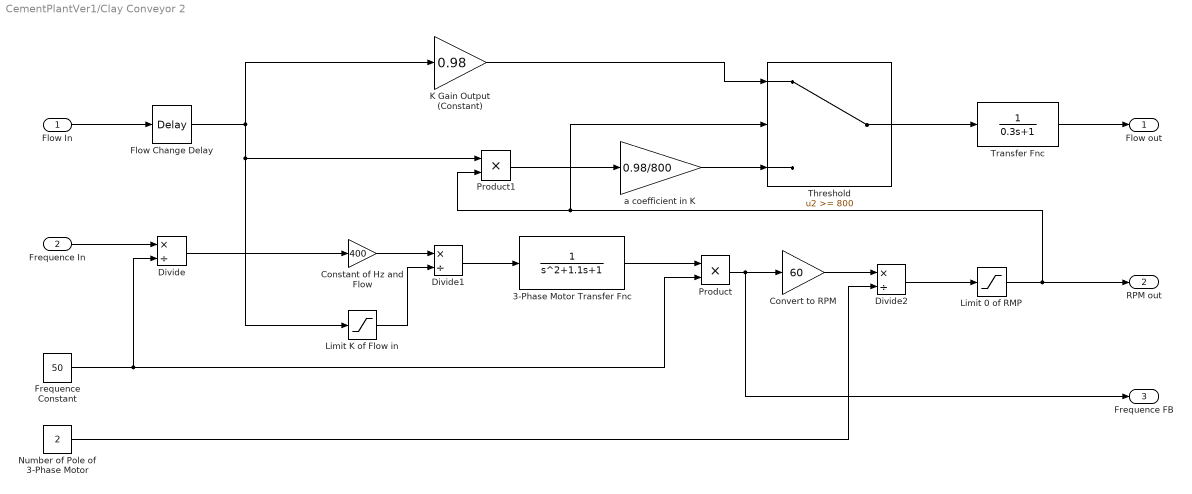
== system CementPlantVer1/Clay Conveyor 2 ==
  Flow In : Inport
  Frequence In : Inport  Port=2
  3-Phase Motor Transfer Fnc : TransferFcn  Denominator=[1 1.1 1]
  Constant of Hz and Flow : Gain  Gain=400
  Convert to RPM : Gain  Gain=60
  Divide : Product  Inputs=*/
  Divide1 : Product  Inputs=*/
  Divide2 : Product  Inputs=*/
  Flow Change Delay : TransportDelay  DelayTime=0.5
  Frequence Constant : Constant  Value=50
  K Gain Output (Constant) : Gain  Gain=0.98
  Limit 0 of RMP : Saturate  UpperLimit=inf  LowerLimit=0
  Limit K of Flow in : Saturate  UpperLimit=inf  LowerLimit=400
  Number of Pole of 3-Phase Motor : Constant  Value=2
  Product : Product
  Product1 : Product
  Threshold : Switch  Threshold=800
  Transfer Fnc : TransferFcn  Denominator=[0.3 1]
  a coefficient in K : Gain  Gain=0.98/800
  Flow out : Outport
  RPM out : Outport  Port=2
  Frequence FB : Outport  Port=3
  wires:
  Constant of Hz and Flow/1 -> Divide1/1
  Limit K of Flow in/1 -> Divide1/2
  Divide1/1 -> 3-Phase Motor Transfer Fnc/1
  Limit 0 of RMP/1 -> RPM out/1, Threshold/2, Product1/2
  Flow In/1 -> Flow Change Delay/1
  Flow Change Delay/1 -> Product1/1, Limit K of Flow in/1, K Gain Output (Constant)/1
  K Gain Output (Constant)/1 -> Threshold/1
  Frequence In/1 -> Divide/1
  Divide/1 -> Constant of Hz and Flow/1
  Frequence Constant/1 -> Product/2, Divide/2
  3-Phase Motor Transfer Fnc/1 -> Product/1
  Product/1 -> Frequence FB/1, Convert to RPM/1
  Convert to RPM/1 -> Divide2/1
  Divide2/1 -> Limit 0 of RMP/1
  Number of Pole of 3-Phase Motor/1 -> Divide2/2
  Threshold/1 -> Transfer Fnc/1
  Transfer Fnc/1 -> Flow out/1
  Product1/1 -> a coefficient in K/1
  a coefficient in K/1 -> Threshold/3

== system CementPlantVer1/Clay Crusher 1 ==
  Flow In : Inport
  Frequence In : Inport  Port=2
  3-Phase Motor Transfer Fnc : TransferFcn  Denominator=[1 2.5 1]
  Constant of Hz and Flow : Gain  Gain=400
  Convert to RPM : Gain  Gain=60
  Divide : Product  Inputs=*/
  Divide1 : Product  Inputs=*/
  Divide2 : Product  Inputs=*/
  Flow Change Delay : TransportDelay  DelayTime=0.5
  Frequence Constant : Constant  Value=50
  K Gain Output (Constant) : Gain
  Limit 0 of RMP : Saturate  UpperLimit=inf  LowerLimit=0
  Limit K of Flow in : Saturate  UpperLimit=inf  LowerLimit=400
  Number of Pole of 3-Phase Motor : Constant  Value=2
  Product : Product
  Product1 : Product
  Threshold : Switch  Threshold=800
  Transfer Fnc : TransferFcn  Denominator=[0.1 1]
  a coefficient in K : Gain  Gain=1/800
  Flow out : Outport
  Frequence FB : Outport  Port=2
  wires:
  Constant of Hz and Flow/1 -> Divide1/1
  Limit K of Flow in/1 -> Divide1/2
  Divide1/1 -> 3-Phase Motor Transfer Fnc/1
  Limit 0 of RMP/1 -> Threshold/2, Product1/2
  Flow In/1 -> Flow Change Delay/1
  Flow Change Delay/1 -> Product1/1, Limit K of Flow in/1, K Gain Output (Constant)/1
  K Gain Output (Constant)/1 -> Threshold/1
  Frequence In/1 -> Divide/1
  Divide/1 -> Constant of Hz and Flow/1
  Frequence Constant/1 -> Product/2, Divide/2
  3-Phase Motor Transfer Fnc/1 -> Product/1
  Product/1 -> Frequence FB/1, Convert to RPM/1
  Convert to RPM/1 -> Divide2/1
  Divide2/1 -> Limit 0 of RMP/1
  Number of Pole of 3-Phase Motor/1 -> Divide2/2
  Threshold/1 -> Transfer Fnc/1
  Transfer Fnc/1 -> Flow out/1
  Product1/1 -> a coefficient in K/1
  a coefficient in K/1 -> Threshold/3

== system CementPlantVer1/Clay Storage ==
  Qin : Inport
  Qout : Inport  Port=2
  A : Gain  Gain=1/(3.14*3*3)
  Convert h to s : Constant  Value=3600
  Density of Clay : Constant  Value=DensityOfMaterial
  Divide : Product  Inputs=*/
  Divide1 : Product  Inputs=*/
  High Operator : RelationalOperator  OutDataTypeStr=boolean  RndMeth=Simplest
  High Level Set (m) : Constant  Value=HighLevelSet
  Low Operator : RelationalOperator  Operator=<=  OutDataTypeStr=boolean  RndMeth=Simplest
  Low Level Set (m) : Constant  Value=LowLevelSet
  Output Coefficient : Gain  Gain=OutputGain
  Saturation Limit : Saturate  UpperLimit=20  LowerLimit=0
  Sum1 : Sum  Inputs=|+-
  Transfer Fnc of Silo : TransferFcn  Denominator=[1 0]
  Level : Outport
  High : Outport  Port=2
  Low : Outport  Port=3
  wires:
  A/1 -> Output Coefficient/1
  Low Operator/1 -> Low/1
  High Level Set (m)/1 -> High Operator/2
  Low Level Set (m)/1 -> Low Operator/2
  Density of Clay/1 -> Divide/2
  Output Coefficient/1 -> Saturation Limit/1
  Convert h to s/1 -> Divide1/2
  Transfer Fnc of Silo/1 -> A/1
  Divide1/1 -> Transfer Fnc of Silo/1
  High Operator/1 -> High/1
  Saturation Limit/1 -> Level/1, Low Operator/1, High Operator/1
  Divide/1 -> Divide1/1
  Sum1/1 -> Divide/1
  Qin/1 -> Sum1/1
  Qout/1 -> Sum1/2

== system CementPlantVer1/Clay Valve 1 ==
  Opening Percent : Inport
  Enable : Inport  Port=2
  Level of Silo : Inport  Port=3
  Constant : Constant  Value=0
  Delay 1s : TransportDelay
  Divide : Product  Inputs=*/
  Maxium Value : Constant  Value=100
  Output Coefficient : Gain  Gain=OutputGain
  Switch : Switch  Threshold=1
  Switch1 : Switch  Criteria=u2 > Threshold
  Transfer Fnc : TransferFcn  Denominator=[20 1]
  Flow : Outport
  wires:
  Transfer Fnc/1 -> Delay 1s/1
  Enable/1 -> Switch/2
  Constant/1 -> Switch/3, Switch1/3
  Opening Percent/1 -> Divide/1
  Divide/1 -> Switch/1
  Maxium Value/1 -> Divide/2
  Output Coefficient/1 -> Flow/1
  Delay 1s/1 -> Output Coefficient/1
  Switch1/1 -> Transfer Fnc/1
  Switch/1 -> Switch1/1
  Level of Silo/1 -> Switch1/2

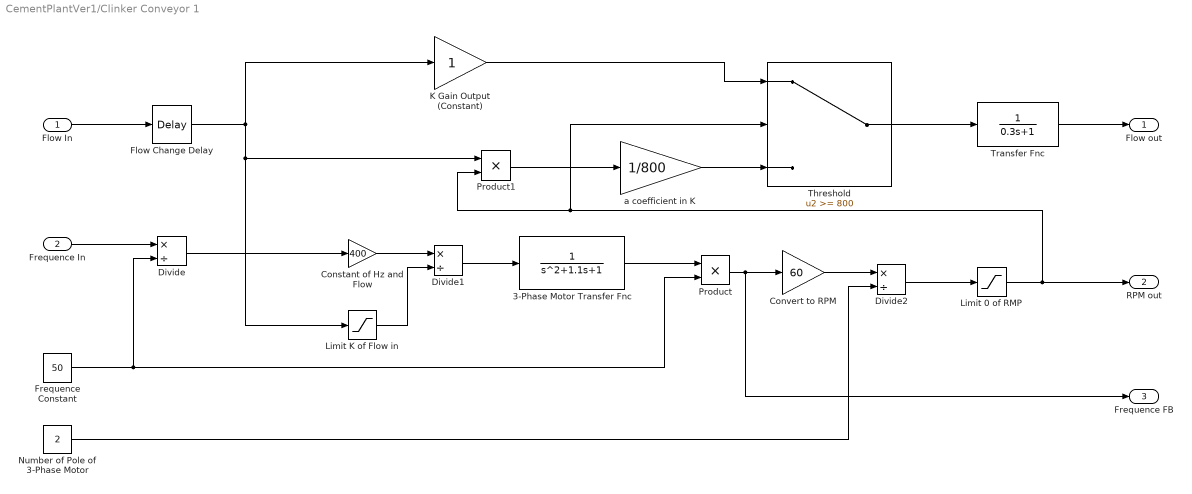
== system CementPlantVer1/Clinker Conveyor 1 ==
  Flow In : Inport
  Frequence In : Inport  Port=2
  3-Phase Motor Transfer Fnc : TransferFcn  Denominator=[1 1.1 1]
  Constant of Hz and Flow : Gain  Gain=400
  Convert to RPM : Gain  Gain=60
  Divide : Product  Inputs=*/
  Divide1 : Product  Inputs=*/
  Divide2 : Product  Inputs=*/
  Flow Change Delay : TransportDelay  DelayTime=0.5
  Frequence Constant : Constant  Value=50
  K Gain Output (Constant) : Gain
  Limit 0 of RMP : Saturate  UpperLimit=inf  LowerLimit=0
  Limit K of Flow in : Saturate  UpperLimit=inf  LowerLimit=400
  Number of Pole of 3-Phase Motor : Constant  Value=2
  Product : Product
  Product1 : Product
  Threshold : Switch  Threshold=800
  Transfer Fnc : TransferFcn  Denominator=[0.3 1]
  a coefficient in K : Gain  Gain=1/800
  Flow out : Outport
  RPM out : Outport  Port=2
  Frequence FB : Outport  Port=3
  wires:
  Constant of Hz and Flow/1 -> Divide1/1
  Limit K of Flow in/1 -> Divide1/2
  Divide1/1 -> 3-Phase Motor Transfer Fnc/1
  Limit 0 of RMP/1 -> RPM out/1, Threshold/2, Product1/2
  Flow In/1 -> Flow Change Delay/1
  Flow Change Delay/1 -> Product1/1, Limit K of Flow in/1, K Gain Output (Constant)/1
  K Gain Output (Constant)/1 -> Threshold/1
  Frequence In/1 -> Divide/1
  Divide/1 -> Constant of Hz and Flow/1
  Frequence Constant/1 -> Product/2, Divide/2
  3-Phase Motor Transfer Fnc/1 -> Product/1
  Product/1 -> Frequence FB/1, Convert to RPM/1
  Convert to RPM/1 -> Divide2/1
  Divide2/1 -> Limit 0 of RMP/1
  Number of Pole of 3-Phase Motor/1 -> Divide2/2
  Threshold/1 -> Transfer Fnc/1
  Transfer Fnc/1 -> Flow out/1
  Product1/1 -> a coefficient in K/1
  a coefficient in K/1 -> Threshold/3

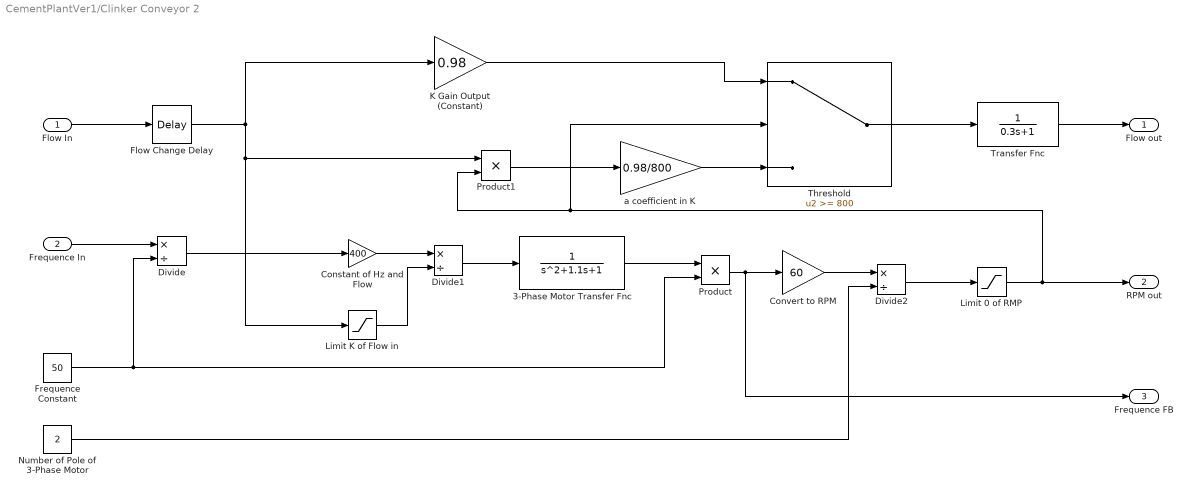
== system CementPlantVer1/Clinker Conveyor 2 ==
  Flow In : Inport
  Frequence In : Inport  Port=2
  3-Phase Motor Transfer Fnc : TransferFcn  Denominator=[1 1.1 1]
  Constant of Hz and Flow : Gain  Gain=400
  Convert to RPM : Gain  Gain=60
  Divide : Product  Inputs=*/
  Divide1 : Product  Inputs=*/
  Divide2 : Product  Inputs=*/
  Flow Change Delay : TransportDelay  DelayTime=0.5
  Frequence Constant : Constant  Value=50
  K Gain Output (Constant) : Gain  Gain=0.98
  Limit 0 of RMP : Saturate  UpperLimit=inf  LowerLimit=0
  Limit K of Flow in : Saturate  UpperLimit=inf  LowerLimit=400
  Number of Pole of 3-Phase Motor : Constant  Value=2
  Product : Product
  Product1 : Product
  Threshold : Switch  Threshold=800
  Transfer Fnc : TransferFcn  Denominator=[0.3 1]
  a coefficient in K : Gain  Gain=0.98/800
  Flow out : Outport
  RPM out : Outport  Port=2
  Frequence FB : Outport  Port=3
  wires:
  Constant of Hz and Flow/1 -> Divide1/1
  Limit K of Flow in/1 -> Divide1/2
  Divide1/1 -> 3-Phase Motor Transfer Fnc/1
  Limit 0 of RMP/1 -> RPM out/1, Threshold/2, Product1/2
  Flow In/1 -> Flow Change Delay/1
  Flow Change Delay/1 -> Product1/1, Limit K of Flow in/1, K Gain Output (Constant)/1
  K Gain Output (Constant)/1 -> Threshold/1
  Frequence In/1 -> Divide/1
  Divide/1 -> Constant of Hz and Flow/1
  Frequence Constant/1 -> Product/2, Divide/2
  3-Phase Motor Transfer Fnc/1 -> Product/1
  Product/1 -> Frequence FB/1, Convert to RPM/1
  Convert to RPM/1 -> Divide2/1
  Divide2/1 -> Limit 0 of RMP/1
  Number of Pole of 3-Phase Motor/1 -> Divide2/2
  Threshold/1 -> Transfer Fnc/1
  Transfer Fnc/1 -> Flow out/1
  Product1/1 -> a coefficient in K/1
  a coefficient in K/1 -> Threshold/3

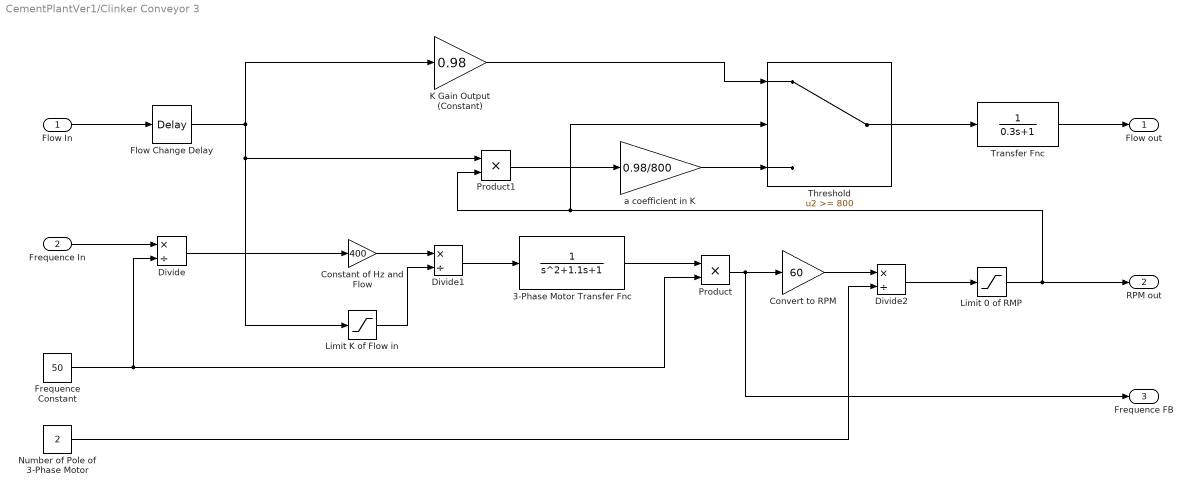
== system CementPlantVer1/Clinker Conveyor 3 ==
  Flow In : Inport
  Frequence In : Inport  Port=2
  3-Phase Motor Transfer Fnc : TransferFcn  Denominator=[1 1.1 1]
  Constant of Hz and Flow : Gain  Gain=400
  Convert to RPM : Gain  Gain=60
  Divide : Product  Inputs=*/
  Divide1 : Product  Inputs=*/
  Divide2 : Product  Inputs=*/
  Flow Change Delay : TransportDelay  DelayTime=0.5
  Frequence Constant : Constant  Value=50
  K Gain Output (Constant) : Gain  Gain=0.98
  Limit 0 of RMP : Saturate  UpperLimit=inf  LowerLimit=0
  Limit K of Flow in : Saturate  UpperLimit=inf  LowerLimit=400
  Number of Pole of 3-Phase Motor : Constant  Value=2
  Product : Product
  Product1 : Product
  Threshold : Switch  Threshold=800
  Transfer Fnc : TransferFcn  Denominator=[0.3 1]
  a coefficient in K : Gain  Gain=0.98/800
  Flow out : Outport
  RPM out : Outport  Port=2
  Frequence FB : Outport  Port=3
  wires:
  Constant of Hz and Flow/1 -> Divide1/1
  Limit K of Flow in/1 -> Divide1/2
  Divide1/1 -> 3-Phase Motor Transfer Fnc/1
  Limit 0 of RMP/1 -> RPM out/1, Threshold/2, Product1/2
  Flow In/1 -> Flow Change Delay/1
  Flow Change Delay/1 -> Product1/1, Limit K of Flow in/1, K Gain Output (Constant)/1
  K Gain Output (Constant)/1 -> Threshold/1
  Frequence In/1 -> Divide/1
  Divide/1 -> Constant of Hz and Flow/1
  Frequence Constant/1 -> Product/2, Divide/2
  3-Phase Motor Transfer Fnc/1 -> Product/1
  Product/1 -> Frequence FB/1, Convert to RPM/1
  Convert to RPM/1 -> Divide2/1
  Divide2/1 -> Limit 0 of RMP/1
  Number of Pole of 3-Phase Motor/1 -> Divide2/2
  Threshold/1 -> Transfer Fnc/1
  Transfer Fnc/1 -> Flow out/1
  Product1/1 -> a coefficient in K/1
  a coefficient in K/1 -> Threshold/3

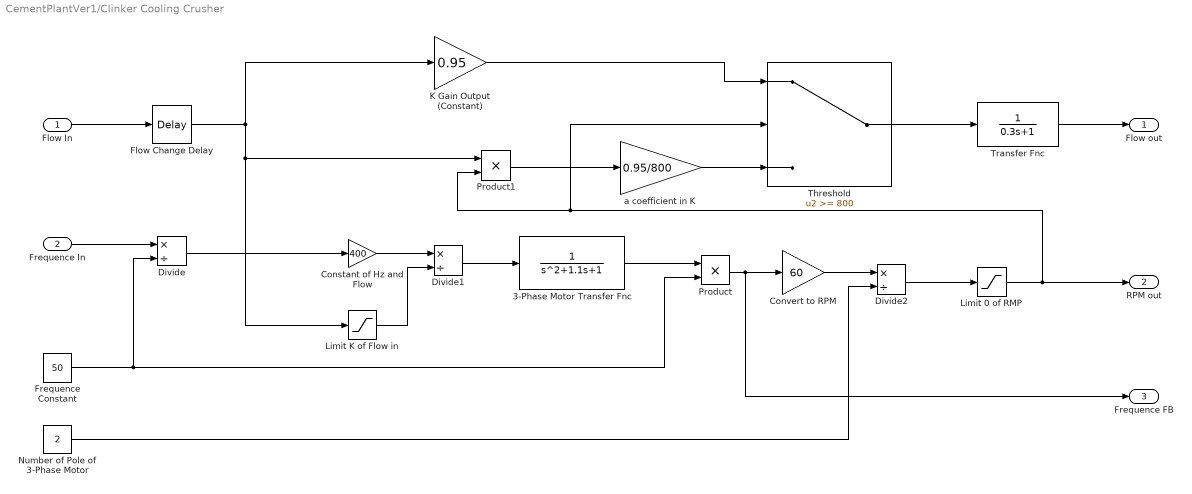
== system CementPlantVer1/Clinker Cooling Crusher ==
  Flow In : Inport
  Frequence In : Inport  Port=2
  3-Phase Motor Transfer Fnc : TransferFcn  Denominator=[1 1.1 1]
  Constant of Hz and Flow : Gain  Gain=400
  Convert to RPM : Gain  Gain=60
  Divide : Product  Inputs=*/
  Divide1 : Product  Inputs=*/
  Divide2 : Product  Inputs=*/
  Flow Change Delay : TransportDelay  DelayTime=0.5
  Frequence Constant : Constant  Value=50
  K Gain Output (Constant) : Gain  Gain=0.95
  Limit 0 of RMP : Saturate  UpperLimit=inf  LowerLimit=0
  Limit K of Flow in : Saturate  UpperLimit=inf  LowerLimit=400
  Number of Pole of 3-Phase Motor : Constant  Value=2
  Product : Product
  Product1 : Product
  Threshold : Switch  Threshold=800
  Transfer Fnc : TransferFcn  Denominator=[0.3 1]
  a coefficient in K : Gain  Gain=0.95/800
  Flow out : Outport
  RPM out : Outport  Port=2
  Frequence FB : Outport  Port=3
  wires:
  Constant of Hz and Flow/1 -> Divide1/1
  Limit K of Flow in/1 -> Divide1/2
  Divide1/1 -> 3-Phase Motor Transfer Fnc/1
  Limit 0 of RMP/1 -> RPM out/1, Threshold/2, Product1/2
  Flow In/1 -> Flow Change Delay/1
  Flow Change Delay/1 -> Product1/1, Limit K of Flow in/1, K Gain Output (Constant)/1
  K Gain Output (Constant)/1 -> Threshold/1
  Frequence In/1 -> Divide/1
  Divide/1 -> Constant of Hz and Flow/1
  Frequence Constant/1 -> Product/2, Divide/2
  3-Phase Motor Transfer Fnc/1 -> Product/1
  Product/1 -> Frequence FB/1, Convert to RPM/1
  Convert to RPM/1 -> Divide2/1
  Divide2/1 -> Limit 0 of RMP/1
  Number of Pole of 3-Phase Motor/1 -> Divide2/2
  Threshold/1 -> Transfer Fnc/1
  Transfer Fnc/1 -> Flow out/1
  Product1/1 -> a coefficient in K/1
  a coefficient in K/1 -> Threshold/3

== system CementPlantVer1/Clinker Fan 1 ==
  Input Frequence : Inport
  Motor Enable : Inport  Port=2
  Constant : Constant  Value=0
  Divide : Product  Inputs=*/
  Frequency Constant : Constant  Value=50
  Frequency Constant FB : Constant  Value=50
  Motor Transfer Function : TransferFcn  Denominator=[1 3.156 1]
  Output coefficient : Constant  Value=1350
  Product : Product
  Product1 : Product
  Saturation : Saturate  UpperLimit=50  LowerLimit=0
  Switch : Switch  Threshold=1
  Output RPM : Outport
  Output Frequence : Outport  Port=2
  wires:
  Product/1 -> Output RPM/1
  Frequency Constant FB/1 -> Product1/2
  Output coefficient/1 -> Product/1
  Frequency Constant/1 -> Divide/2
  Motor Transfer Function/1 -> Product/2, Product1/1
  Input Frequence/1 -> Divide/1
  Saturation/1 -> Output Frequence/1
  Product1/1 -> Saturation/1
  Divide/1 -> Switch/1
  Switch/1 -> Motor Transfer Function/1
  Motor Enable/1 -> Switch/2
  Constant/1 -> Switch/3
